simulink model "files_write_read_delete_test"  (R2022a)
settings: Solver=FixedStepAuto  StartTime=0.0  StopTime=inf  FixedStep=0.001  RelTol=1e-3
undefined symbols (not defined in the file): CR, d, LF
libraries: dspstat3 x24, simulink x3, instrumentlib x2, matrix_library x1, slrealtimeutilitieslib x1, commcrc2 x1
settings Model: Creator=DeveloperY  LastModifiedBy=DeveloperY

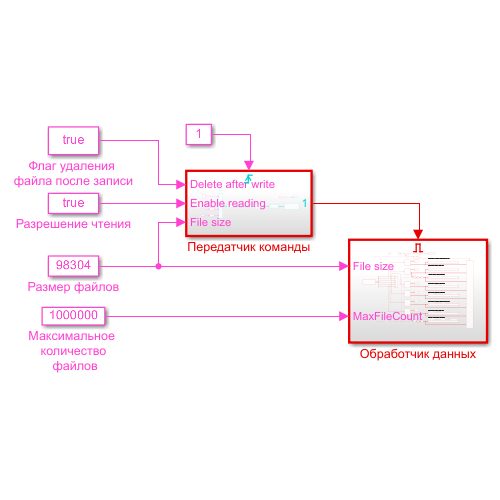
[thumbnail: Simulink's stored preview of the top-level diagram]
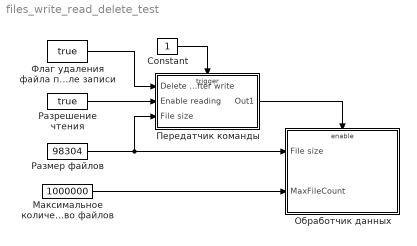
== system files_write_read_delete_test ==
  Constant : Constant
  Максимальное количество файлов : Constant  Value=1000000  OutDataTypeStr=uint32
  Обработчик данных : Subsystem  TreatAsAtomicUnit=on
  Передатчик команды : Subsystem  TreatAsAtomicUnit=on
  Размер файлов : Constant  Value=98304  OutDataTypeStr=uint32
  Разрешение чтения : Constant  Value=true
  Флаг удаления файла после записи : Constant  Value=true
  wires:
  Constant/1 -> Передатчик команды/Trigger
  Флаг удаления файла после записи/1 -> Передатчик команды/1(Delete after write)
  Размер файлов/1 -> Обработчик данных/1(File size), Передатчик команды/3(File size)
  Максимальное количество файлов/1 -> Обработчик данных/2(MaxFileCount)
  Разрешение чтения/1 -> Передатчик команды/2(Enable reading)
  Передатчик команды/1(Out1) -> Обработчик данных/Enable

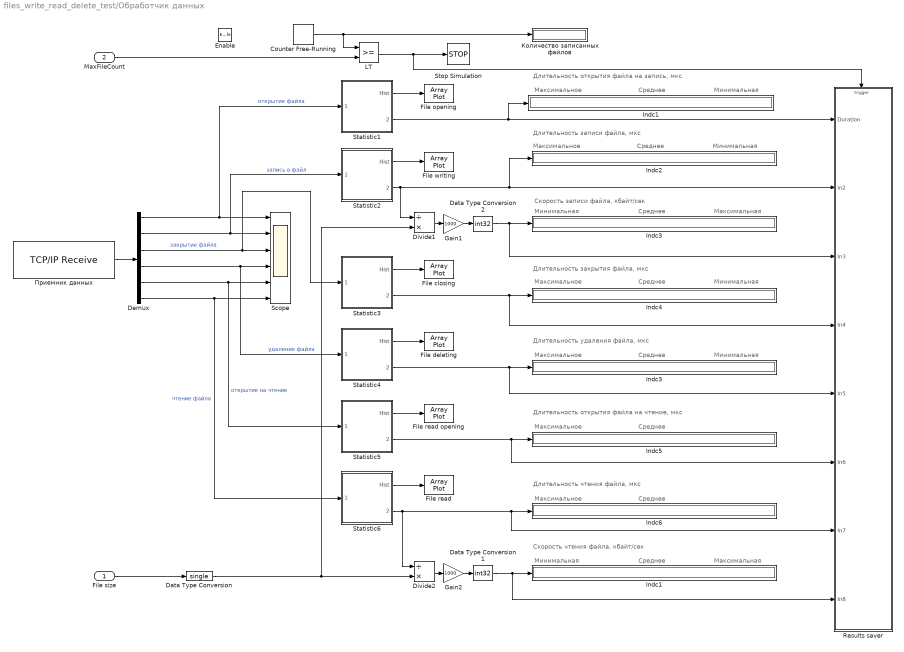
== system files_write_read_delete_test/Обработчик данных ==
  note: Длительность открытия файла на запись, мкс
  note: Минимальная
  note: Среднее
  note: Максимальное
  note: Минимальная
  note: Максимальная
  note: Максимальное
  note: Среднее
  note: Длительность записи файла, мкс
  note: Минимальная
  note: Скорость записи файла, кбайт/сек
  note: Среднее
  note: Минимальная
  note: Максимальное
  note: Среднее
  note: Длительность закрытия файла, мкс
  note: Длительность удаления файла, мкс
  note: Среднее
  note: Минимальная
  note: Максимальное
  note: Максимальное
  note: Среднее
  note: Длительность открытия файла на чтение, мкс
  note: Максимальное
  note: Среднее
  note: Длительность чтения файла, мкс
  note: Минимальная
  note: Максимальная
  note: Среднее
  note: Скорость чтения файла, кбайт/сек
  File size : Inport
  MaxFileCount : Inport  Port=2
  Enable : EnablePort
   Indc{1..6} (6 alike) : Display
  Counter Free-Running : simulink/Sources/Counter Free-Running  NumBits=32  tsamp=-1
  Data Type Conversion : DataTypeConversion  OutDataTypeStr=single  SaturateOnIntegerOverflow=off  RndMeth=Floor
  Data Type Conversion1 : DataTypeConversion  OutDataTypeStr=int32  SaturateOnIntegerOverflow=off  RndMeth=Floor
  Data Type Conversion2 : DataTypeConversion  OutDataTypeStr=int32  SaturateOnIntegerOverflow=off  RndMeth=Floor
  Demux : Demux  Outputs=6
  Divide1 : Product  Inputs=/*  OutDataTypeStr=single
  Divide2 : Product  Inputs=/*  OutDataTypeStr=single
  File closing : ArrayPlot  WindowPosition=[1308.000000,91.000000,562.000000,274.000000,]  Visible=on  ScopeFrameLocation=window  SampleIncrement=0.5  YScale=Log  PlotType=Stairs  AxesScaling=Manual  YLimits=[-24.5,200]  ShowLegend=on
  File deleting : ArrayPlot  WindowPosition=[1308.000000,91.000000,562.000000,274.000000,]  Visible=on  ScopeFrameLocation=window  SampleIncrement=0.5  YScale=Log  PlotType=Stairs  AxesScaling=Manual  YLimits=[-24.5,200]  ShowLegend=on
  File opening : ArrayPlot  WindowPosition=[1311.000000,673.000000,562.000000,326.000000,]  Visible=on  ScopeFrameLocation=window  SampleIncrement=0.5  YScale=Log  PlotType=Stairs  AxesScaling=Manual  YLimits=[-24.5,200]  ShowLegend=on
  File read : ArrayPlot  WindowPosition=[1308.000000,91.000000,562.000000,274.000000,]  Visible=on  ScopeFrameLocation=window  SampleIncrement=0.5  YScale=Log  PlotType=Stairs  AxesScaling=Manual  YLimits=[-24.5,200]  ShowLegend=on
  File read opening : ArrayPlot  WindowPosition=[1308.000000,91.000000,562.000000,274.000000,]  Visible=on  ScopeFrameLocation=window  SampleIncrement=0.5  YScale=Log  PlotType=Stairs  AxesScaling=Manual  YLimits=[-24.5,200]  ShowLegend=on
  File writing : ArrayPlot  WindowPosition=[1310.000000,375.000000,562.000000,288.000000,]  Visible=on  ScopeFrameLocation=window  SampleIncrement=300  YScale=Log  PlotType=Stairs  AxesScaling=Manual  YLimits=[-24.5,200]  ShowLegend=on
  Gain1 : Gain  Gain=1000
  Gain2 : Gain  Gain=1000
  Indc1 : Display
  Indc3 : Display
  LT : RelationalOperator  OutDataTypeStr=boolean  RndMeth=Simplest  InputSameDT=off
  Results saver : Subsystem  TreatAsAtomicUnit=on
  Scope : Scope  NumInputPorts=6
  Statistic1 : Subsystem
  Statistic2 : Subsystem
  Statistic3 : Subsystem
  Statistic4 : Subsystem
  Statistic5 : Subsystem
  Statistic6 : Subsystem
  Stop Simulation : Stop
  Количество записанных файлов : Display
  Приемник данных : instrumentlib/TCP//IP Receive  Host=192.168.3.1  Port=3333  DataSize=[6]  DataType=ASCII  ASCIIFormatting=%d,%d,%d,%d,%d,%d  Terminator=CR/LF  CustomTerminator=10  ByteOrder=big-endian  EnableBlockingMode=on  Timeout=1  SampleTime=-1  SimulateUsing=Interpreted execution
  wires:
  Demux/3 -> Scope/3, Statistic3/1(Samples)  "закрытие файла"
  Demux/2 -> Scope/2, Statistic2/1(Samples)  "запись в файл"
  Demux/1 -> Scope/1, Statistic1/1(Samples)  "открытие файла"
  Приемник данных/1 -> Demux/1
  Counter Free-Running/1 -> LT/1, Количество записанных файлов/1
  Statistic1/1(Hist) -> File opening/1
  Statistic1/2(Duration) -> " Indc1"/1, Results saver/1(Duration)
  Divide1/1 -> Gain1/1
  Data Type Conversion2/1 -> Results saver/3(In3), Indc3/1
  File size/1 -> Data Type Conversion/1
  Gain1/1 -> Data Type Conversion2/1
  Statistic2/2(Duration) -> Divide1/1, " Indc2"/1, Results saver/2(In2)
  Statistic3/2(Duration) -> Results saver/4(In4), " Indc4"/1
  Statistic2/1(Hist) -> File writing/1
  Statistic3/1(Hist) -> File closing/1
  Demux/4 -> Scope/4, Statistic4/1(Samples)  "удаление файла"
  Statistic4/1(Hist) -> File deleting/1
  Statistic4/2(Duration) -> Results saver/5(In5), " Indc3"/1
  MaxFileCount/1 -> LT/2
  LT/1 -> Stop Simulation/1, Results saver/Trigger
  Data Type Conversion/1 -> Divide1/2, Divide2/2
  Demux/5 -> Scope/5, Statistic5/1(Samples)  "открытие на чтение"
  Demux/6 -> Scope/6, Statistic6/1(Samples)  "чтение файла"
  Statistic5/1(Hist) -> File read opening/1
  Statistic5/2(Duration) -> Results saver/6(In6), " Indc5"/1
  Statistic6/2(Duration) -> Divide2/1, Results saver/7(In7), " Indc6"/1
  Statistic6/1(Hist) -> File read/1
  Data Type Conversion1/1 -> Results saver/8(In8), Indc1/1
  Gain2/1 -> Data Type Conversion1/1
  Divide2/1 -> Gain2/1

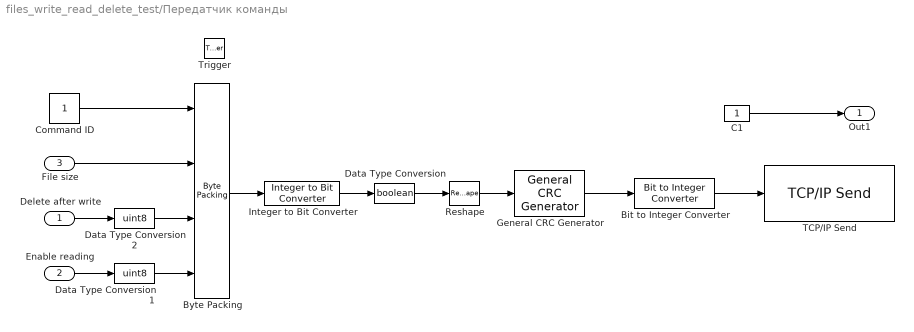
== system files_write_read_delete_test/Передатчик команды ==
  Delete after write : Inport
  Enable reading : Inport  Port=2
  File size : Inport  Port=3
  Trigger : TriggerPort  VariantControl=(inherit)  InitialTriggerSignalState=zero
  " C1" : Constant  OutDataTypeStr=uint32
  Bit to Integer Converter : simulink/Logic and Bit Operations/Bit to Integer Converter  nbits=8  bitOrder=MSB first  signedOutputValues=Unsigned  outDtype=Inherit via internal rule  outDtypeSigned=Inherit via internal rule
      settings: SourceProductBaseCode=SL
  Byte Packing : slrealtimeutilitieslib/Byte Packing  MaskPackedDataType=uint8  MaskUnpackedDataTypes={'uint32','uint32','uint8', 'uint8' }  MaskAlignment=1
  Command ID : Constant  OutDataTypeStr=uint32
  Data Type Conversion : DataTypeConversion  OutDataTypeStr=boolean  SaturateOnIntegerOverflow=off  RndMeth=Floor
  Data Type Conversion1 : DataTypeConversion  OutDataTypeStr=uint8  SaturateOnIntegerOverflow=off  RndMeth=Floor
  Data Type Conversion2 : DataTypeConversion  OutDataTypeStr=uint8  SaturateOnIntegerOverflow=off  RndMeth=Floor
  General CRC Generator : commcrc2/General CRC Generator  genPoly='z^16 + z^12 + z^5 + 1'  iniStates=0  directMethod=off  reflectInputBytes=off  reflectChecksums=off  finalXOR=0  numChecksums=1
      settings: SourceProductBaseCode=CM
  Integer to Bit Converter : simulink/Logic and Bit Operations/Integer to Bit Converter  nbits=8  signedInputValues=Unsigned  bitOrder=MSB first  outDtype=Inherit via internal rule
      settings: SourceProductBaseCode=SL
  Reshape : Reshape  OutputDimensionality=Customize  OutputDimensions=[80,1]
  TCP/IP Send : instrumentlib/TCP//IP Send  Host=192.168.3.1  Port=3333  ByteOrder=big-endian  EnableBlockingMode=off  Timeout=0.1  TransferDelay=on  SimulateUsing=Interpreted execution
  Out1 : Outport
  wires:
  Command ID/1 -> Byte Packing/1
  File size/1 -> Byte Packing/2
  Delete after write/1 -> Data Type Conversion2/1
  Data Type Conversion2/1 -> Byte Packing/3
  Integer to Bit Converter/1 -> Data Type Conversion/1
  Data Type Conversion/1 -> Reshape/1
  Reshape/1 -> General CRC Generator/1
  General CRC Generator/1 -> Bit to Integer Converter/1
  Bit to Integer Converter/1 -> TCP/IP Send/1
  Byte Packing/1 -> Integer to Bit Converter/1
  Data Type Conversion1/1 -> Byte Packing/4
  Enable reading/1 -> Data Type Conversion1/1
  " C1"/1 -> Out1/1

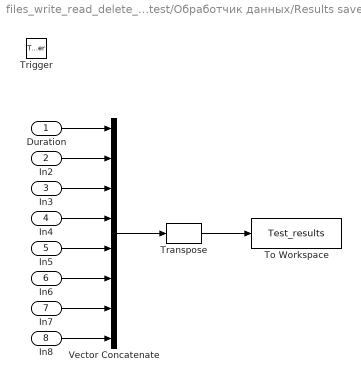
== system files_write_read_delete_test/Обработчик данных/Results saver ==
  Duration : Inport
  In2 : Inport  Port=2
  In3 : Inport  Port=3
  In4 : Inport  Port=4
  In5 : Inport  Port=5
  In6 : Inport  Port=6
  In7 : Inport  Port=7
  In8 : Inport  Port=8
  Trigger : TriggerPort  VariantControl=(inherit)  InitialTriggerSignalState=zero
  To Workspace : ToWorkspace  VariableName=Test_results  SampleTime=-1
  Transpose : matrix_library/Transpose
      settings: SourceProductBaseCode=SL
  Vector Concatenate : Concatenate  NumInputs=8  Mode=Multidimensional array  ConcatenateDimension=2
  wires:
  In2/1 -> Vector Concatenate/2
  Duration/1 -> Vector Concatenate/1
  In3/1 -> Vector Concatenate/3
  Vector Concatenate/1 -> Transpose/1
  In5/1 -> Vector Concatenate/5
  In4/1 -> Vector Concatenate/4
  Transpose/1 -> To Workspace/1
  In6/1 -> Vector Concatenate/6
  In7/1 -> Vector Concatenate/7
  In8/1 -> Vector Concatenate/8

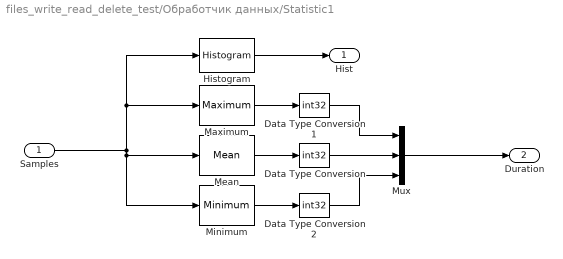
== system files_write_read_delete_test/Обработчик данных/Statistic1 ==
  Samples : Inport
  Data Type Conversion : DataTypeConversion  OutDataTypeStr=int32  SaturateOnIntegerOverflow=off  RndMeth=Floor
  Data Type Conversion1 : DataTypeConversion  OutDataTypeStr=int32  SaturateOnIntegerOverflow=off  RndMeth=Floor
  Data Type Conversion2 : DataTypeConversion  OutDataTypeStr=int32  SaturateOnIntegerOverflow=off  RndMeth=Floor
  Histogram : dspstat3/Histogram  umin=0  umax=1000000  nbins=100  operateOver=Entire input  Dimension=1  normalized=off  run=on  reset=on  trigtype=None  colComp=on  roundingMode=Floor  overflowMode=off
      settings: SourceProductBaseCode=DS
  Maximum : dspstat3/Maximum  operation=maximum  fcn=Running  indexBase=One  operateOver=Specified dimension  Dimension=1  reset=None  roiEnable=off  roiType=Rectangles  roiPortion=Entire ROI  roiOutput=Individual statistics for each ROI  roiFlag=off  roundingMode=Floor  overflowMode=off  accumDataTypeStr=Inherit: Same as product output  accumLastDataTypeStr=Inherit: Same as product output
  Mean : dspstat3/Mean  run=on  reset_popup=None  directionMode=Entire input  dimension=1  roiEnable=off  roiType=Rectangles  roiPortion=Entire ROI  roiOutput=Individual statistics for each ROI  roiFlag=off  roundingMode=Floor  overflowMode=off  outputDataTypeStr=Inherit: Same as accumulator  outputMin=[]  outputMax=[]  outputLastDataTypeStr=Inherit: Same as accumulator
  Minimum : dspstat3/Minimum  operation=minimum  fcn=Running  indexBase=One  operateOver=Entire input  Dimension=1  reset=None  roiEnable=off  roiType=Rectangles  roiPortion=Entire ROI  roiOutput=Individual statistics for each ROI  roiFlag=off  roundingMode=Floor  overflowMode=off
      settings: SourceProductBaseCode=DS
  Mux : Mux  Inputs=3
  Hist : Outport
  Duration : Outport  Port=2
  wires:
  Histogram/1 -> Hist/1
  Maximum/1 -> Data Type Conversion1/1
  Minimum/1 -> Data Type Conversion2/1
  Samples/1 -> Minimum/1, Mean/1, Maximum/1, Histogram/1
  Mean/1 -> Data Type Conversion/1
  Data Type Conversion/1 -> Mux/2
  Data Type Conversion1/1 -> Mux/1
  Data Type Conversion2/1 -> Mux/3
  Mux/1 -> Duration/1

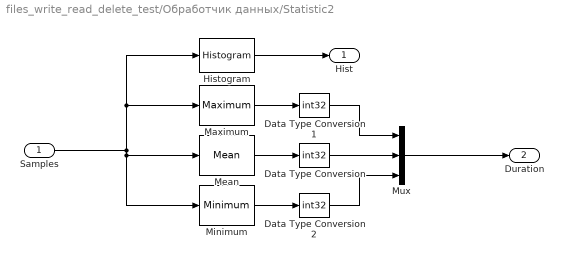
== system files_write_read_delete_test/Обработчик данных/Statistic2 ==
  Samples : Inport
  Data Type Conversion : DataTypeConversion  OutDataTypeStr=int32  SaturateOnIntegerOverflow=off  RndMeth=Floor
  Data Type Conversion1 : DataTypeConversion  OutDataTypeStr=int32  SaturateOnIntegerOverflow=off  RndMeth=Floor
  Data Type Conversion2 : DataTypeConversion  OutDataTypeStr=int32  SaturateOnIntegerOverflow=off  RndMeth=Floor
  Histogram : dspstat3/Histogram  umin=0  umax=30000  nbins=100  operateOver=Entire input  Dimension=1  normalized=off  run=on  reset=on  trigtype=None  colComp=on  roundingMode=Floor  overflowMode=off
      settings: SourceProductBaseCode=DS
  Maximum : dspstat3/Maximum  operation=maximum  fcn=Running  indexBase=One  operateOver=Specified dimension  Dimension=1  reset=None  roiEnable=off  roiType=Rectangles  roiPortion=Entire ROI  roiOutput=Individual statistics for each ROI  roiFlag=off  roundingMode=Floor  overflowMode=off  accumDataTypeStr=Inherit: Same as product output  accumLastDataTypeStr=Inherit: Same as product output
  Mean : dspstat3/Mean  run=on  reset_popup=None  directionMode=Entire input  dimension=1  roiEnable=off  roiType=Rectangles  roiPortion=Entire ROI  roiOutput=Individual statistics for each ROI  roiFlag=off  roundingMode=Floor  overflowMode=off  outputDataTypeStr=Inherit: Same as accumulator  outputMin=[]  outputMax=[]  outputLastDataTypeStr=Inherit: Same as accumulator
  Minimum : dspstat3/Minimum  operation=minimum  fcn=Running  indexBase=One  operateOver=Entire input  Dimension=1  reset=None  roiEnable=off  roiType=Rectangles  roiPortion=Entire ROI  roiOutput=Individual statistics for each ROI  roiFlag=off  roundingMode=Floor  overflowMode=off
      settings: SourceProductBaseCode=DS
  Mux : Mux  Inputs=3
  Hist : Outport
  Duration : Outport  Port=2
  wires:
  Histogram/1 -> Hist/1
  Maximum/1 -> Data Type Conversion1/1
  Minimum/1 -> Data Type Conversion2/1
  Samples/1 -> Minimum/1, Mean/1, Maximum/1, Histogram/1
  Mean/1 -> Data Type Conversion/1
  Data Type Conversion/1 -> Mux/2
  Data Type Conversion1/1 -> Mux/1
  Data Type Conversion2/1 -> Mux/3
  Mux/1 -> Duration/1

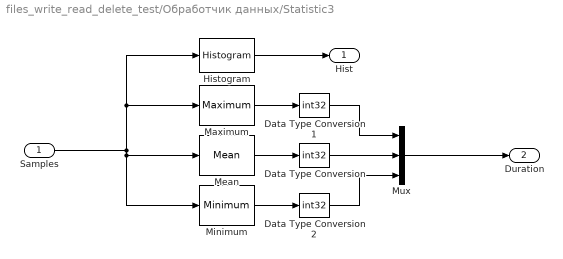
== system files_write_read_delete_test/Обработчик данных/Statistic3 ==
  Samples : Inport
  Data Type Conversion : DataTypeConversion  OutDataTypeStr=int32  SaturateOnIntegerOverflow=off  RndMeth=Floor
  Data Type Conversion1 : DataTypeConversion  OutDataTypeStr=int32  SaturateOnIntegerOverflow=off  RndMeth=Floor
  Data Type Conversion2 : DataTypeConversion  OutDataTypeStr=int32  SaturateOnIntegerOverflow=off  RndMeth=Floor
  Histogram : dspstat3/Histogram  umin=0  umax=50  nbins=100  operateOver=Entire input  Dimension=1  normalized=off  run=on  reset=on  trigtype=None  colComp=on  roundingMode=Floor  overflowMode=off
      settings: SourceProductBaseCode=DS
  Maximum : dspstat3/Maximum  operation=maximum  fcn=Running  indexBase=One  operateOver=Specified dimension  Dimension=1  reset=None  roiEnable=off  roiType=Rectangles  roiPortion=Entire ROI  roiOutput=Individual statistics for each ROI  roiFlag=off  roundingMode=Floor  overflowMode=off  accumDataTypeStr=Inherit: Same as product output  accumLastDataTypeStr=Inherit: Same as product output
  Mean : dspstat3/Mean  run=on  reset_popup=None  directionMode=Entire input  dimension=1  roiEnable=off  roiType=Rectangles  roiPortion=Entire ROI  roiOutput=Individual statistics for each ROI  roiFlag=off  roundingMode=Floor  overflowMode=off  outputDataTypeStr=Inherit: Same as accumulator  outputMin=[]  outputMax=[]  outputLastDataTypeStr=Inherit: Same as accumulator
  Minimum : dspstat3/Minimum  operation=minimum  fcn=Running  indexBase=One  operateOver=Entire input  Dimension=1  reset=None  roiEnable=off  roiType=Rectangles  roiPortion=Entire ROI  roiOutput=Individual statistics for each ROI  roiFlag=off  roundingMode=Floor  overflowMode=off
      settings: SourceProductBaseCode=DS
  Mux : Mux  Inputs=3
  Hist : Outport
  Duration : Outport  Port=2
  wires:
  Histogram/1 -> Hist/1
  Maximum/1 -> Data Type Conversion1/1
  Minimum/1 -> Data Type Conversion2/1
  Samples/1 -> Minimum/1, Mean/1, Maximum/1, Histogram/1
  Mean/1 -> Data Type Conversion/1
  Data Type Conversion/1 -> Mux/2
  Data Type Conversion1/1 -> Mux/1
  Data Type Conversion2/1 -> Mux/3
  Mux/1 -> Duration/1

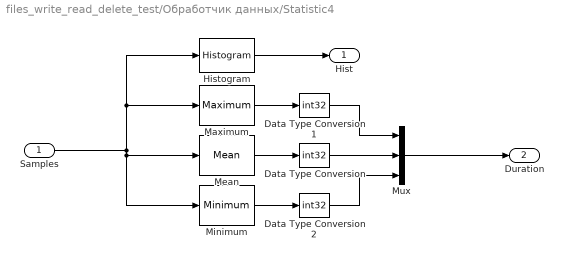
== system files_write_read_delete_test/Обработчик данных/Statistic4 ==
  Samples : Inport
  Data Type Conversion : DataTypeConversion  OutDataTypeStr=int32  SaturateOnIntegerOverflow=off  RndMeth=Floor
  Data Type Conversion1 : DataTypeConversion  OutDataTypeStr=int32  SaturateOnIntegerOverflow=off  RndMeth=Floor
  Data Type Conversion2 : DataTypeConversion  OutDataTypeStr=int32  SaturateOnIntegerOverflow=off  RndMeth=Floor
  Histogram : dspstat3/Histogram  umin=0  umax=50  nbins=100  operateOver=Entire input  Dimension=1  normalized=off  run=on  reset=on  trigtype=None  colComp=on  roundingMode=Floor  overflowMode=off
      settings: SourceProductBaseCode=DS
  Maximum : dspstat3/Maximum  operation=maximum  fcn=Running  indexBase=One  operateOver=Specified dimension  Dimension=1  reset=None  roiEnable=off  roiType=Rectangles  roiPortion=Entire ROI  roiOutput=Individual statistics for each ROI  roiFlag=off  roundingMode=Floor  overflowMode=off  accumDataTypeStr=Inherit: Same as product output  accumLastDataTypeStr=Inherit: Same as product output
  Mean : dspstat3/Mean  run=on  reset_popup=None  directionMode=Entire input  dimension=1  roiEnable=off  roiType=Rectangles  roiPortion=Entire ROI  roiOutput=Individual statistics for each ROI  roiFlag=off  roundingMode=Floor  overflowMode=off  outputDataTypeStr=Inherit: Same as accumulator  outputMin=[]  outputMax=[]  outputLastDataTypeStr=Inherit: Same as accumulator
  Minimum : dspstat3/Minimum  operation=minimum  fcn=Running  indexBase=One  operateOver=Entire input  Dimension=1  reset=None  roiEnable=off  roiType=Rectangles  roiPortion=Entire ROI  roiOutput=Individual statistics for each ROI  roiFlag=off  roundingMode=Floor  overflowMode=off
      settings: SourceProductBaseCode=DS
  Mux : Mux  Inputs=3
  Hist : Outport
  Duration : Outport  Port=2
  wires:
  Histogram/1 -> Hist/1
  Maximum/1 -> Data Type Conversion1/1
  Minimum/1 -> Data Type Conversion2/1
  Samples/1 -> Minimum/1, Mean/1, Maximum/1, Histogram/1
  Mean/1 -> Data Type Conversion/1
  Data Type Conversion/1 -> Mux/2
  Data Type Conversion1/1 -> Mux/1
  Data Type Conversion2/1 -> Mux/3
  Mux/1 -> Duration/1

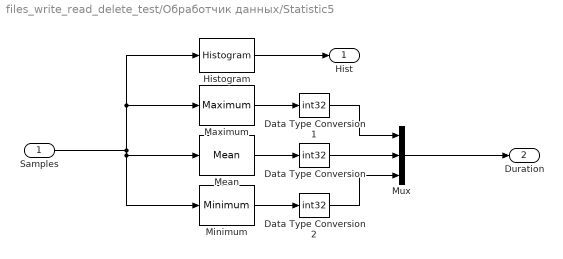
== system files_write_read_delete_test/Обработчик данных/Statistic5 ==
  Samples : Inport
  Data Type Conversion : DataTypeConversion  OutDataTypeStr=int32  SaturateOnIntegerOverflow=off  RndMeth=Floor
  Data Type Conversion1 : DataTypeConversion  OutDataTypeStr=int32  SaturateOnIntegerOverflow=off  RndMeth=Floor
  Data Type Conversion2 : DataTypeConversion  OutDataTypeStr=int32  SaturateOnIntegerOverflow=off  RndMeth=Floor
  Histogram : dspstat3/Histogram  umin=0  umax=50  nbins=100  operateOver=Entire input  Dimension=1  normalized=off  run=on  reset=on  trigtype=None  colComp=on  roundingMode=Floor  overflowMode=off
      settings: SourceProductBaseCode=DS
  Maximum : dspstat3/Maximum  operation=maximum  fcn=Running  indexBase=One  operateOver=Specified dimension  Dimension=1  reset=None  roiEnable=off  roiType=Rectangles  roiPortion=Entire ROI  roiOutput=Individual statistics for each ROI  roiFlag=off  roundingMode=Floor  overflowMode=off  accumDataTypeStr=Inherit: Same as product output  accumLastDataTypeStr=Inherit: Same as product output
  Mean : dspstat3/Mean  run=on  reset_popup=None  directionMode=Entire input  dimension=1  roiEnable=off  roiType=Rectangles  roiPortion=Entire ROI  roiOutput=Individual statistics for each ROI  roiFlag=off  roundingMode=Floor  overflowMode=off  outputDataTypeStr=Inherit: Same as accumulator  outputMin=[]  outputMax=[]  outputLastDataTypeStr=Inherit: Same as accumulator
  Minimum : dspstat3/Minimum  operation=minimum  fcn=Running  indexBase=One  operateOver=Entire input  Dimension=1  reset=None  roiEnable=off  roiType=Rectangles  roiPortion=Entire ROI  roiOutput=Individual statistics for each ROI  roiFlag=off  roundingMode=Floor  overflowMode=off
      settings: SourceProductBaseCode=DS
  Mux : Mux  Inputs=3
  Hist : Outport
  Duration : Outport  Port=2
  wires:
  Histogram/1 -> Hist/1
  Maximum/1 -> Data Type Conversion1/1
  Minimum/1 -> Data Type Conversion2/1
  Samples/1 -> Minimum/1, Mean/1, Maximum/1, Histogram/1
  Mean/1 -> Data Type Conversion/1
  Data Type Conversion/1 -> Mux/2
  Data Type Conversion1/1 -> Mux/1
  Data Type Conversion2/1 -> Mux/3
  Mux/1 -> Duration/1

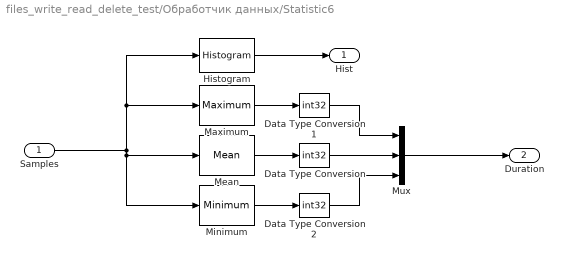
== system files_write_read_delete_test/Обработчик данных/Statistic6 ==
  Samples : Inport
  Data Type Conversion : DataTypeConversion  OutDataTypeStr=int32  SaturateOnIntegerOverflow=off  RndMeth=Floor
  Data Type Conversion1 : DataTypeConversion  OutDataTypeStr=int32  SaturateOnIntegerOverflow=off  RndMeth=Floor
  Data Type Conversion2 : DataTypeConversion  OutDataTypeStr=int32  SaturateOnIntegerOverflow=off  RndMeth=Floor
  Histogram : dspstat3/Histogram  umin=0  umax=50  nbins=100  operateOver=Entire input  Dimension=1  normalized=off  run=on  reset=on  trigtype=None  colComp=on  roundingMode=Floor  overflowMode=off
      settings: SourceProductBaseCode=DS
  Maximum : dspstat3/Maximum  operation=maximum  fcn=Running  indexBase=One  operateOver=Specified dimension  Dimension=1  reset=None  roiEnable=off  roiType=Rectangles  roiPortion=Entire ROI  roiOutput=Individual statistics for each ROI  roiFlag=off  roundingMode=Floor  overflowMode=off  accumDataTypeStr=Inherit: Same as product output  accumLastDataTypeStr=Inherit: Same as product output
  Mean : dspstat3/Mean  run=on  reset_popup=None  directionMode=Entire input  dimension=1  roiEnable=off  roiType=Rectangles  roiPortion=Entire ROI  roiOutput=Individual statistics for each ROI  roiFlag=off  roundingMode=Floor  overflowMode=off  outputDataTypeStr=Inherit: Same as accumulator  outputMin=[]  outputMax=[]  outputLastDataTypeStr=Inherit: Same as accumulator
  Minimum : dspstat3/Minimum  operation=minimum  fcn=Running  indexBase=One  operateOver=Entire input  Dimension=1  reset=None  roiEnable=off  roiType=Rectangles  roiPortion=Entire ROI  roiOutput=Individual statistics for each ROI  roiFlag=off  roundingMode=Floor  overflowMode=off
      settings: SourceProductBaseCode=DS
  Mux : Mux  Inputs=3
  Hist : Outport
  Duration : Outport  Port=2
  wires:
  Histogram/1 -> Hist/1
  Maximum/1 -> Data Type Conversion1/1
  Minimum/1 -> Data Type Conversion2/1
  Samples/1 -> Minimum/1, Mean/1, Maximum/1, Histogram/1
  Mean/1 -> Data Type Conversion/1
  Data Type Conversion/1 -> Mux/2
  Data Type Conversion1/1 -> Mux/1
  Data Type Conversion2/1 -> Mux/3
  Mux/1 -> Duration/1
